simulink model "pindreg"  (Simulink 7.4)
settings: Solver=ode45  StartTime=0.0  StopTime=30  RelTol=1e-3
values from neighbouring files (symbols this model uses):
  Bs = 1.748817703686052e-04    (= 0.000174881770369)    [pindregStart.m]
  g = 9.816    [pindregStart.m]    (also in tilstandsREG.m)
  initU = 1.7    [pindregStart.m]    (also in tilstandsREG.m)
  Js = 2.686970843428432e-04    (= 0.000268697084343)    [pindregStart.m]    (also in tilstandsREG.m)
  Km = 0.022141706562986    (= 0.022141706563)    [pindregStart.m]    (also in tilstandsREG.m)
  la = 0.3384    [pindregStart.m]    (also in tilstandsREG.m)
  lp = 1.1509    [pindregStart.m]    (also in tilstandsREG.m)
  ma = 0.298    [pindregStart.m]    (also in tilstandsREG.m)
  N = 12/40    (= 0.3)    [pindregStart.m]    (also in tilstandsREG.m)
  Rm = 0.807790757873553    (= 0.807790757874)    [pindregStart.m]    (also in tilstandsREG.m)
  tauf = 0.064    [pindregStart.m]    (also in tilstandsREG.m)
libraries: vrlib x3, simulink x1
settings Model: Creator=Skov  LastModifiedBy=Skov

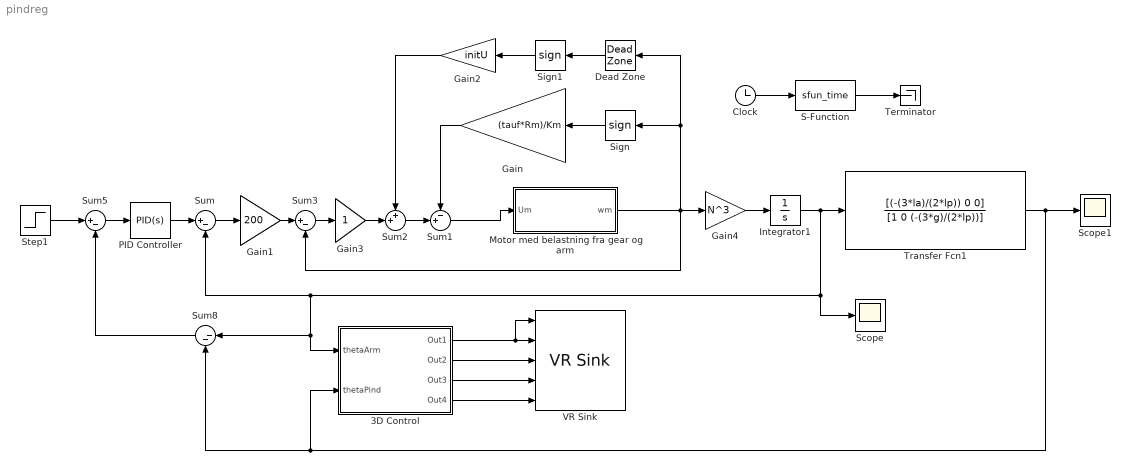
== system pindreg ==
  3D Control : Subsystem
  Clock : Clock
      settings: Decimation=10
  Dead Zone : DeadZone  LowerValue=-0.1  UpperValue=0.1  SaturateOnIntegerOverflow=on
  Gain : Gain  Gain=(tauf*Rm)/Km  ParameterDataType=fixdt(1, 16)  ParameterScaling=2^0  OutDataType=fixdt(1, 16)  OutScaling=2^0
  Gain1 : Gain  Gain=200  ParameterDataType=fixdt(1, 16)  ParameterScaling=2^0  OutDataType=fixdt(1, 16)  OutScaling=2^0
  Gain2 : Gain  Gain=initU  ParameterDataType=fixdt(1, 16)  ParameterScaling=2^0  OutDataType=fixdt(1, 16)  OutScaling=2^0
  Gain3 : Gain  ParameterDataType=fixdt(1, 16)  ParameterScaling=2^0  OutDataType=fixdt(1, 16)  OutScaling=2^0
  Gain4 : Gain  Gain=N^3  ParameterDataType=fixdt(1, 16)  ParameterScaling=2^0  OutDataType=fixdt(1, 16)  OutScaling=2^0
  Integrator1 : Integrator
  Motor med belastning fra gear og arm : Subsystem
  PID Controller : simulink/Continuous/PID Controller  DialogController=pidpack.PIDConfig.pidDDGCreate  DialogControllerArgs=DataTag0  SystemSampleTime=-1  Controller=PID  TimeDomain=Continuous-time  SampleTime=1  IntegratorMethod=Forward Euler  FilterMethod=Forward Euler  Form=Parallel  P=100  I=20  D=1000  N=100  InitialConditionSource=internal  InitialConditionForIntegrator=0  InitialConditionForFilter=0  ExternalReset=none  LimitOutput=off  UpperSaturationLimit=inf  LowerSaturationLimit=-inf  LinearizeAsGain=off  AntiWindupMode=none  Kb=1  TrackingMode=off  Kt=1  PParamMin=[]  PParamMax=[]  IParamMin=[]  IParamMax=[]  DParamMin=[]  DParamMax=[]  NParamMin=[]  NParamMax=[]  KbParamMin=[]  KbParamMax=[]  KtParamMin=[]  KtParamMax=[]  POutMin=[]  POutMax=[]  IOutMin=[]  IOutMax=[]  DOutMin=[]  DOutMax=[]  NOutMin=[]  NOutMax=[]  KbOutMin=[]  KbOutMax=[]  KtOutMin=[]  KtOutMax=[]  IntegratorOutMin=[]  IntegratorOutMax=[]  FilterOutMin=[]  FilterOutMax=[]  SumOutMin=[]  SumOutMax=[]  SumI1OutMin=[]  SumI1OutMax=[]  SumI2OutMin=[]  SumI2OutMax=[]  SumI3OutMin=[]  SumI3OutMax=[]  SumDOutMin=[]  SumDOutMax=[]  SaturationOutMin=[]  SaturationOutMax=[]  IntegratorContinuousStateAttributes=''  IntegratorStateMustResolveToSignalObject=off  IntegratorRTWStateStorageClass=Auto  FilterContinuousStateAttributes=''  FilterStateMustResolveToSignalObject=off  FilterRTWStateStorageClass=Auto
  S-Function : S-Function  FunctionName=sfun_time  EnableBusSupport=off
  Scope : Scope
      settings: YMin=-0.65  YMax=0.05
  Scope1 : Scope
      settings: YMin=-0.4  YMax=0.45
  Sign : Signum  SampleTime=0.01
  Sign1 : Signum
  Step1 : Step  Time=3  After=pi/8  SampleTime=0
  Sum : Sum  Inputs=|+-  OutDataType=fixdt(1, 16)  OutScaling=2^0
  Sum1 : Sum  Inputs=-+|  OutDataType=fixdt(1, 16)  OutScaling=2^0
  Sum2 : Sum  Inputs=++|  OutDataType=fixdt(1, 16)  OutScaling=2^0
  Sum3 : Sum  Inputs=|+-  OutDataType=fixdt(1, 16)  OutScaling=2^0
  Sum5 : Sum  Inputs=|+-  OutDataType=fixdt(1, 16)  OutScaling=2^0
  Sum8 : Sum  Inputs=|--  OutDataType=fixdt(1, 16)  OutScaling=2^0
  Terminator : Terminator
  Transfer Fcn1 : TransferFcn  Numerator=[(-(3*la)/(2*lp)) 0 0]  Denominator=[1 0 (-(3*g)/(2*lp))]
  VR Sink : vrlib/VR Sink  InstantiateOnLoad=on  SampleTime=0.02  ViewEnable=on  RemoteChange=off  RemoteView=on  FieldsWritten=Ball.rotation.4.1.double#Arm.rotation.4.1.double#Pind.translation.3.1.double#AP.translation.3.1.double#Pind.rotation.4.1.double  WorldFileName=VRML1.WRL  AutoView=off  VideoDimensions=[]  FigureProperties="{'Position', 'Name', 'Viewpoint', 'CameraBound', 'CameraDirection', 'CameraPosition', 'CameraUpVector', 'ZoomFactor', 'Antialiasing', 'Headlight', 'Lighting', 'NavPanel', 'StatusBar', 'ToolBar', 'Textures', 'Transparency', 'Wireframe', 'NavZones', 'NavMode', 'NavSpeed', 'Record2DCompressMethod', 'Record2DCompressQuality', 'Record2D', 'Record2DFileName', 'Record2DFPS'; [7.9000000000000000e+01   1.6000000000000000e+02   7.7300000000000000e+02   5.4700000000000000e+02], '', '', 'on', [0.0000000000000000e+00   3.1410759078128292e-02  -9.9950656036573160e-01], [0.0000000000000000e+00   0.0000000000000000e+00   1.0000000000000000e+01], [0.0000000000000000e+00   9.9950656036573160e-01   3.1410759078128292e-02], [5.1315811823070645e-01], 'off', 'on', 'on', 'halfbar', 'on', 'on', 'on', 'on', 'off', 'off', 'fly', 'normal', 'auto', [7.5000000000000000e+01], 'off', '%f_anim_%n.avi', [1.5000000000000000e+01]}"
  wires:
  Sign/1 -> Gain/1
  Gain/1 -> Sum1/1
  Sum3/1 -> Gain3/1
  Gain4/1 -> Integrator1/1
  Integrator1/1 -> Transfer Fcn1/1, Sum/2, 3D Control/1(thetaArm), Sum8/1, Scope/1
  Gain1/1 -> Sum3/1
  Sum1/1 -> Motor med belastning fra gear og arm/1(Um)
  Sum/1 -> Gain1/1
  S-Function/1 -> Terminator/1
  Clock/1 -> S-Function/1
  Sum2/1 -> Sum1/2
  Dead Zone/1 -> Sign1/1
  Sign1/1 -> Gain2/1
  Gain3/1 -> Sum2/2
  Gain2/1 -> Sum2/1
  Step1/1 -> Sum5/1
  Sum8/1 -> Sum5/2
  PID Controller/1 -> Sum/1
  Sum5/1 -> PID Controller/1
  Transfer Fcn1/1 -> Sum8/2, 3D Control/2(thetaPind), Scope1/1
  Motor med belastning fra gear og arm/1(wm) -> Gain4/1, Sign/1, Dead Zone/1, Sum3/2
  3D Control/1(Out1) -> VR Sink/1, VR Sink/2
  3D Control/2(Out2) -> VR Sink/3
  3D Control/3(Out3) -> VR Sink/4
  3D Control/4(Out4) -> VR Sink/5

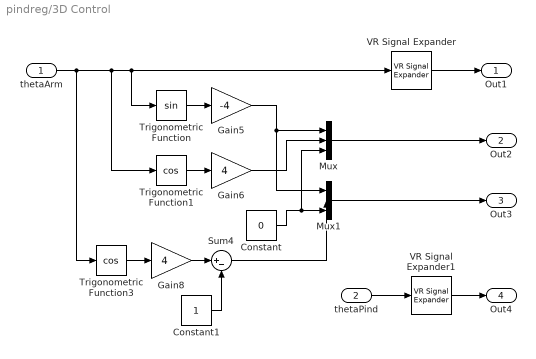
== system pindreg/3D Control ==
  thetaArm : Inport  OutDataType=fixdt(1, 16)  OutScaling=2^0
  thetaPind : Inport  Port=2  OutDataType=fixdt(1, 16)  OutScaling=2^0
  Constant : Constant  Value=0  OutDataType=fixdt(1, 16)  OutScaling=2^0
  Constant1 : Constant  OutDataType=fixdt(1, 16)  OutScaling=2^0
  Gain5 : Gain  Gain=-4  ParameterDataType=fixdt(1, 16)  ParameterScaling=2^0  OutDataType=fixdt(1, 16)  OutScaling=2^0
  Gain6 : Gain  Gain=4  ParameterDataType=fixdt(1, 16)  ParameterScaling=2^0  OutDataType=fixdt(1, 16)  OutScaling=2^0
  Gain8 : Gain  Gain=4  ParameterDataType=fixdt(1, 16)  ParameterScaling=2^0  OutDataType=fixdt(1, 16)  OutScaling=2^0
  Mux : Mux  Inputs=3
  Mux1 : Mux  Inputs=3
  Sum4 : Sum  Inputs=|+-  OutDataType=fixdt(1, 16)  OutScaling=2^0
  Trigonometric Function : Trigonometry
  Trigonometric Function1 : Trigonometry  Operator=cos
  Trigonometric Function3 : Trigonometry  Operator=cos
  VR Signal Expander : vrlib/VR Signal Expander  SystemSampleTime=-1  outwidth=4  outidx=[4]
  VR Signal Expander1 : vrlib/VR Signal Expander  SystemSampleTime=-1  outwidth=4  outidx=[4]
  Out1 : Outport  OutDataType=fixdt(1, 16)  OutScaling=2^0
  Out2 : Outport  Port=2  OutDataType=fixdt(1, 16)  OutScaling=2^0
  Out3 : Outport  Port=3  OutDataType=fixdt(1, 16)  OutScaling=2^0
  Out4 : Outport  Port=4  OutDataType=fixdt(1, 16)  OutScaling=2^0
  wires:
  VR Signal Expander/1 -> Out1/1
  Trigonometric Function/1 -> Gain5/1
  Gain5/1 -> Mux/1, Mux1/1
  Trigonometric Function1/1 -> Gain6/1
  Gain6/1 -> Mux/2
  Constant/1 -> Mux/3, Mux1/3
  Mux/1 -> Out2/1
  Trigonometric Function3/1 -> Gain8/1
  Gain8/1 -> Sum4/1
  Constant1/1 -> Sum4/2
  Sum4/1 -> Mux1/2
  Mux1/1 -> Out3/1
  VR Signal Expander1/1 -> Out4/1
  thetaPind/1 -> VR Signal Expander1/1
  thetaArm/1 -> VR Signal Expander/1, Trigonometric Function/1, Trigonometric Function1/1, Trigonometric Function3/1

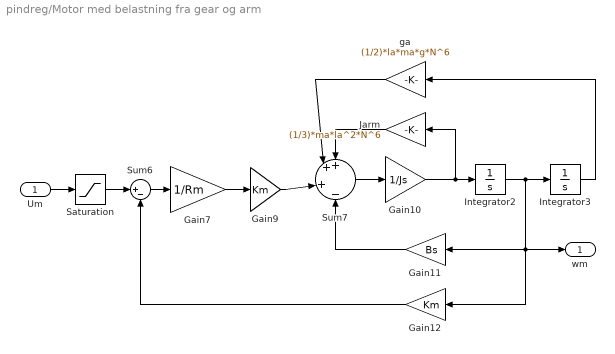
== system pindreg/Motor med belastning fra gear og arm ==
  Um : Inport  OutDataType=fixdt(1, 16)  OutScaling=2^0
  Gain10 : Gain  Gain=1/Js  ParameterDataType=fixdt(1, 16)  ParameterScaling=2^0  OutDataType=fixdt(1, 16)  OutScaling=2^0
  Gain11 : Gain  Gain=Bs  ParameterDataType=fixdt(1, 16)  ParameterScaling=2^0  OutDataType=fixdt(1, 16)  OutScaling=2^0
  Gain12 : Gain  Gain=Km  ParameterDataType=fixdt(1, 16)  ParameterScaling=2^0  OutDataType=fixdt(1, 16)  OutScaling=2^0
  Gain7 : Gain  Gain=1/Rm  ParameterDataType=fixdt(1, 16)  ParameterScaling=2^0  OutDataType=fixdt(1, 16)  OutScaling=2^0
  Gain9 : Gain  Gain=Km  ParameterDataType=fixdt(1, 16)  ParameterScaling=2^0  OutDataType=fixdt(1, 16)  OutScaling=2^0
  Integrator2 : Integrator
  Integrator3 : Integrator
  Jarm : Gain  Gain=(1/3)*ma*la^2*N^6  ParameterDataType=fixdt(1, 16)  ParameterScaling=2^0  OutDataType=fixdt(1, 16)  OutScaling=2^0
  Saturation : Saturate  UpperLimit=13  LowerLimit=-13  OutDataType=fixdt(1, 16)  OutScaling=2^0
  Sum6 : Sum  Inputs=|+-  OutDataType=fixdt(1, 16)  OutScaling=2^0
  Sum7 : Sum  Inputs=++|+|-  OutDataType=fixdt(1, 16)  OutScaling=2^0
  ga : Gain  Gain=(1/2)*la*ma*g*N^6  ParameterDataType=fixdt(1, 16)  ParameterScaling=2^0  OutDataType=fixdt(1, 16)  OutScaling=2^0
  wm : Outport  OutDataType=fixdt(1, 16)  OutScaling=2^0
  wires:
  Sum6/1 -> Gain7/1
  Gain7/1 -> Gain9/1
  Gain10/1 -> Integrator2/1, Jarm/1
  Sum7/1 -> Gain10/1
  Integrator2/1 -> Gain11/1, Gain12/1, wm/1, Integrator3/1
  Gain12/1 -> Sum6/2
  Saturation/1 -> Sum6/1
  Integrator3/1 -> ga/1
  Jarm/1 -> Sum7/1
  ga/1 -> Sum7/2
  Um/1 -> Saturation/1
  Gain9/1 -> Sum7/3
  Gain11/1 -> Sum7/4
